simulink model "controlDeadbeat"  (R2023b)
settings: Solver=VariableStepAuto  StartTime=0.0  StopTime=200  RelTol=1e-3
settings Model: Creator=L03525615  LastModifiedBy=paulverdugo
settings DebuggingCC: UnconnectedInputMsg=warning  UnconnectedOutputMsg=warning  UnconnectedLineMsg=warning
settings ModelReferenceCC: EnableRefExpFcnMdlSchedulingChecks=on
settings RTWCC: DLArmComputeVersion=19.05

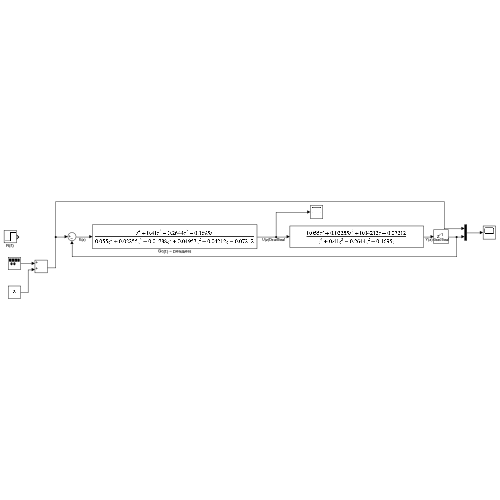
[thumbnail: Simulink's stored preview of the top-level diagram]
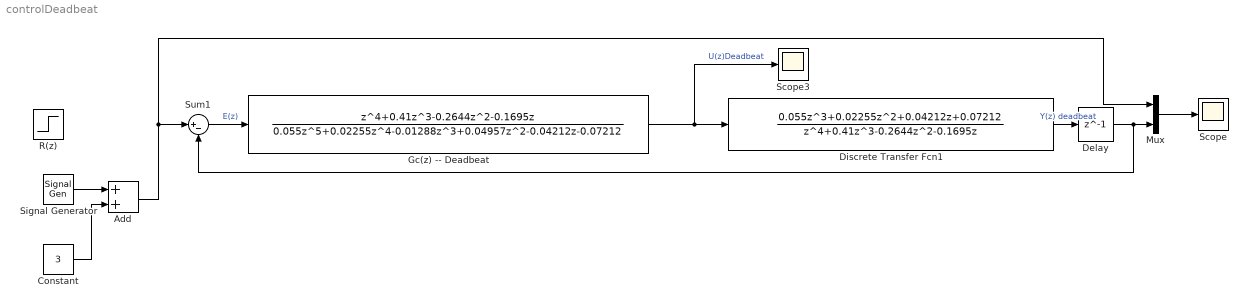
== system controlDeadbeat ==
  Add : Sum
  Constant : Constant  Value=3
  Delay : Delay  DelayLength=1
  Discrete Transfer Fcn1 : DiscreteTransferFcn  Numerator=[0.055 0.02255 0.04212 0.07212]  Denominator=[1 0.41 -0.2644 -0.1695 0 ]  SampleTime=1
  "Gc(z) -- Deadbeat" : DiscreteTransferFcn  Numerator=[1 0.41 -0.2644 -0.1695 0]  Denominator=[0.055 0.02255 -0.01288 0.04957 -0.04212 -0.07212]  SampleTime=1
  Mux : Mux  Inputs=2
  R(z) : Step  Time=10  After=6  SampleTime=0
  Scope : Scope
  Scope3 : Scope
  Signal Generator : SignalGenerator  WaveForm=square  Amplitude=5  Frequency=0.2
  Sum1 : Sum  Inputs=|+-
  wires:
  "Gc(z) -- Deadbeat"/1 -> Discrete Transfer Fcn1/1, Scope3/1  "U(z)Deadbeat"
  Sum1/1 -> "Gc(z) -- Deadbeat"/1  "E(z)"
  Mux/1 -> Scope/1
  Signal Generator/1 -> Add/1
  Constant/1 -> Add/2
  Add/1 -> Mux/1, Sum1/1
  Discrete Transfer Fcn1/1 -> Delay/1  "Y(z) deadbeat"
  Delay/1 -> Sum1/2, Mux/2
